simulink model "transfer_function_calculation"  (R2016a)
settings: Solver=VariableStepAuto  StartTime=0.0  StopTime=5  RelTol=1e-3
values from neighbouring files (symbols this model uses):
  a = .7    (= 0.7)    [PM_1_5MW_syn_27.m]
  Flux = 5.8264    [PM_1_5MW_syn_27.m]
  Id_set = 500    [PM_1_5MW_syn_27.m]
  Iq_set = -2200    [PM_1_5MW_syn_27.m]
  L = .0001    (= 0.0001)    [PM_1_5MW_syn_27.m]
  Ld = 0.001575    [PM_1_5MW_syn_27.m]
  Lq = 0.001575    [PM_1_5MW_syn_27.m]
  mn = 60000    [PM_1_5MW_syn_27.m]
  p = 26    [PM_1_5MW_syn_27.m]
  Rs = 0.000821    [PM_1_5MW_syn_27.m]
  Sollkurve_M_Optimum = [0 57121 101549 158670 228485 310994 406196 514092 634681 767965 810425 823386 ... (13 elements, 13x1)]    [Lookup_M_n.mat]
  Sollkurve_nGen_Optimum = [0 5 7 9 11 12 14 16 18 20 20.07 20.2 ... (13 elements, 13x1)]    [Lookup_M_n.mat]
  Speed_set = w_m    (= 2.10172548525)    [PM_1_5MW_syn_27.m]
  Ts_Power = 5.000000000000000e-06    (= 5e-06)    [PM_1_5MW_syn_27.m]
  Vdc = 1200    [PM_1_5MW_syn_27.m]
  Vh = Vm/6*0    (= 0)    [PM_1_5MW_syn_27.m]
undefined symbols (not defined in the file or in its folder): C2, Esw_Erec, Esw_Off, Esw_On, Page_Temp_C
undefined symbols (not defined in the file): Ts_Control, z
libraries: fl_lib x84, powerlib_meascontrol x58, simulink x56, nesl_utility x36, powerlib x33, simulink_extras x11
(part 2 of 6)

== system transfer_function_calculation/Generator/3 Level Converter2/Loss Calculation ==
  In1 : Inport
  In2 : Inport  Port=2
  In3 : Inport  Port=3
  In4 : Inport  Port=4
  In5 : Inport  Port=5
  In6 : Inport  Port=6
  In7 : Inport  Port=7
  In8 : Inport  Port=8
  In9 : Inport  Port=9
  In10 : Inport  Port=10
  In11 : Inport  Port=11
  In12 : Inport  Port=12
  "A;B;C phase losses " : Scope  NumInputPorts=4
  Leg A1 : Subsystem  mask(Half-Bridge IGBT with thermal model & losses calculation){Ron=1e-3, Rs=1e6, Cs=Inf, Tj_Init=123, PulseDuration=z, Ts=Ts_Power, Ts_Simscape=Ts_Control, IGBT_Rth_jc=0.051/10, IGBT_Cth_j=1.6804*2, IGBT_Vcc_Eon=1200, IGBT_Tj_Eon=[125 150], IGBT_Eon=[150 200 300 450 600 700 900 1000 1200 1400; 150 220 300 500 700 800 1000 1200 1400 1500], IGBT_Ic_Eon=[0 400 800 1600 2400 3200 4000 4800 5600 6400], IGBT_Vcc_Eoff=1200, IGBT_Tj_Eoff=[125 150], IGBT_Eoff=[150 200 400 610 950 1220 1600 2100 2600 3200; 200 350 570 900 1000 1300 1700 2100 2700 3400], IGBT_Ic_Eoff=[0 400 800 1600 2400 3200 4000 4800 5600 6400], IGBT_Tj_OnState=[125 150], IGBT_Vce_OnState=[.5 .81 .9 1 1.5 2 2.5 3 3.5; 0 0.5 .9 1 1.5 2.1 2.6 3.2 3.7], IGBT_Ic_OnState=[0 250 300 400 1300 2600 4200 5600 7200], DIODE_Rth_jc=0.102/10, DIODE_Cth_j=1.3235*2, DIODE_Vcc_Erec=1200, DIODE_Tj_Erec=[125 150], DIODE_Erec=[150 500 650 800 950 1050 1120 1190 1210;350 550 790 950 1100 1200 1270 1320 1350], DIODE_If_Erec=[0 900 1800 2700 3600 4500 5400 6300 7200], DIODE_Tj_OnState=[125 150], DIODE_Vf_OnState=[0 1.0 1.2 1.4 1.7 1.8 1.9 2.2 2.4 2.7;0 1 1.25 1.47 1.72 1.9 2 2.3 2.6 2.8], DIODE_If_OnState=[0 600 1200 1800 2400 3000 3600 4800 6000 7200]}
      mask prompts: Ron "Internal resistance Ron (Ohms):"; Rs "Snubber resistance (Ohms):"; Cs "Snubber capacitance (F):"; Tj_Init "Initial Junction Temperature (degrees Celsius):"; PulseDuration "Pulse Duration for Energy-to-Power conversion (s):"; Ts "Simscape Power Systems Sample Time (as specified in the Powergui) (s):"; Ts_Simscape "Simscape Solver Sample Time (s):"; IGBT_Rth_jc "Junction-to-Case thermal resistance (K/W):"; IGBT_Cth_j "Junction thermal capacitance (Joule/Kelvin):"; IGBT_Vcc_Eon "Vcc (V):"; IGBT_Tj_Eon "Tj  (Celsius):"; IGBT_Eon "Eon (V):"; IGBT_Ic_Eon "Ic (A):"; IGBT_Vcc_Eoff "Vcc (V):"; IGBT_Tj_Eoff "Tj (Celsius):"; IGBT_Eoff "Eoff (V):"; IGBT_Ic_Eoff "Ic (A):"; IGBT_Tj_OnState "Tj (Celsius):"; IGBT_Vce_OnState "Vce (V):"; IGBT_Ic_OnState "Ic (A):"; DIODE_Rth_jc "Junction-to-Case thermal resistance (K/W):"; DIODE_Cth_j "Junction thermal capacitance (Joule/Kelvin):"; DIODE_Vcc_Erec "Vcc (V):"; DIODE_Tj_Erec "Tj  (Celsius):"; DIODE_Erec "Erec (V):"; DIODE_If_Erec "If (A):"; DIODE_Tj_OnState "Tj (Celsius):"; DIODE_Vf_OnState "Vf (V):"; DIODE_If_OnState "If (A):"
      mask help: The half-bridge is modeled by two IGBT/Diode blocks. The upper and lower IGBT/Diode blocks are pulsed from an external pulse generator.
      mask init:
      | BlockName=gcb;
      | Tj0=Tj_Init;
      | 
      | % Add a row with 0 values for Eon and Eoff
      | E0_On=zeros(1,length(IGBT_Eon));
      | Esw_On(:,:,1)=[E0_On;IGBT_Eon(1,:)];
      | Esw_On(:,:,2)=[E0_On;IGBT_Eon(2,:)];
      | E0_Off=zeros(1,length(IGBT_Eoff));
      | Esw_Off(:,:,1)=[E0_Off;IGBT_Eoff(1,:)];
      | Esw_Off(:,:,2)=[E0_Off;IGBT_Eoff(2,:)];
      | 
      | % Create a two-element vector for Vcc (first value = 0)
      | Vcc_Esw_On=[0 IGBT_Vcc_Eon];
      | Vcc_Esw_Off=[0 IGBT_Vcc_Eoff];
      | 
      | % Add a row with 0 values for Erec
      | E0_Erec=zeros(1,length(DIODE_Erec));
      | Esw_Erec(:,:,1)=[E0_Erec;DIODE_Erec(1,:)];
      | Esw_Erec(:,:,2)=[E0_Erec;DIODE_Erec(2,:)];
      | 
      | % Create a two-element vector for Vcc (first value = 0)
      | Vcc_Esw_Erec=[0 DIODE_Vcc_Erec];
      mask DialogControl Container7 Prompt: Specifications
      mask DialogControl Container8 Prompt: Turn-on switching energies
      mask DialogControl Container9 Prompt: Turn-off switching energies
      mask DialogControl Container10 Prompt: On-state characteristics
      mask DialogControl Control4 Prompt: Plot characteristics
      mask DialogControl Control4 Callback:
      | %
      | IGBT_Vcc_Eon = getSPSmaskvalues(gcb,{'IGBT_Vcc_Eon'});
      | IGBT_Tj_Eon  = getSPSmaskvalues(gcb,{'IGBT_Tj_Eon'});
      | IGBT_Eon     = getSPSmaskvalues(gcb,{'IGBT_Eon'});
      | IGBT_Ic_Eon  = getSPSmaskvalues(gcb,{'IGBT_Ic_Eon'});
      | %
      | IGBT_Vcc_Eoff = getSPSmaskvalues(gcb,{'IGBT_Vcc_Eoff'});
      | IGBT_Tj_Eoff  = getSPSmaskvalues(gcb,{'IGBT_Tj_Eoff'});
      | IGBT_Eoff     = getSPSmaskvalues(gcb,{'IGBT_Eoff'});
      | IGBT_Ic_Eoff  = getSPSmaskvalues(gcb,{'IGBT_Ic_Eoff'});
      | %
      | IGBT_Tj_OnState  = getSPSmaskvalues(gcb,{'IGBT_Tj_OnState'});
      | IGBT_Vce_OnState = getSPSmaskvalues(gcb,{'IGBT_Vce_OnState'});
      | IGBT_Ic_OnState  = getSPSmaskvalues(gcb,{'IGBT_Ic_OnState'});
      | %
      | h1=figure;
      | ScreenS=get(0,'Screensize');
      | set(h1,'Position',[ScreenS(3)/60 ScreenS(4)/12 ScreenS(3)/2.4 ScreenS(4)/1.25])
      | subplot(3,1,1)
      | plot(IGBT_Ic_Eon,IGBT_Eon(1,:),'blue', ...
      |      IGBT_Ic_Eon,IGBT_Eon(2,:),'red')
      | legend([num2str(IGBT_Tj_Eon(1)),' deg. C'],[num2str(IGBT_Tj_Eon(2)),' deg. C'],'Location','NorthWest')
      | grid
      | Vcc_Value= num2str(IGBT_Vcc_Eon,'%5.0f');
      | title(['IGBT Turn-on Switching Energy (Vcc= ', Vcc_Value, ' V)' ])
      | ylabel('Eon (mJ)')
      | xlabel('Ic (A)')
      | hold on
      | %
      | subplot(3,1,2)
      | plot(IGBT_Ic_Eoff,IGBT_Eoff(1,:),'blue', ...
      |     IGBT_Ic_Eoff,IGBT_Eoff(2,:),'red')
      | legend([num2str(IGBT_Tj_Eoff(1)),' deg. C'],[num2str(IGBT_Tj_Eoff(2)),' deg. C'],'Location','NorthWest')
      | grid
      | Vcc_Value= num2str(IGBT_Vcc_Eoff,'%5.0f');
      | title(['IGBT Turn-off Switching Energy (Vcc= ', Vcc_Value, ' V)' ])
      | ylabel('Eoff (mJ)')
      | xlabel('Ic (A)')
      | %
      | subplot(3,1,3)
      | plot(IGBT_Vce_OnState(1,:),IGBT_Ic_OnState,'blue', ...
      |     IGBT_Vce_OnState(2,:),IGBT_Ic_OnState,'red')
      | legend([num2str(IGBT_Tj_OnState(1)),' deg. C'],[num2str(IGBT_Tj_OnState(2)),' deg. C'],'Location','NorthWest')
      | grid
      | title('IGBT On-state Characteristics')
      | ylabel('Ic (A)')
      | xlabel('Vce (V)')
      mask DialogControl Container7_copy Prompt: Specifications
      mask DialogControl Container12 Prompt: Reverse recovery energy
      mask DialogControl Container13 Prompt: On-state characteristics
      mask DialogControl Control4_copy Prompt: Plot characteristics
      mask DialogControl Control4_copy Callback:
      | DIODE_If_Erec    = getSPSmaskvalues(gcb,{'DIODE_If_Erec'});
      | DIODE_Erec       = getSPSmaskvalues(gcb,{'DIODE_Erec'});
      | DIODE_Vcc_Erec   = getSPSmaskvalues(gcb,{'DIODE_Vcc_Erec'});
      | DIODE_Vf_OnState = getSPSmaskvalues(gcb,{'DIODE_Vf_OnState'});
      | DIODE_If_OnState = getSPSmaskvalues(gcb,{'DIODE_If_OnState'});
      | 
      | h2=figure;
      | ScreenS=get(0,'Screensize');
      | set(h2,'Position',[ScreenS(3)/2.3 ScreenS(4)/12 ScreenS(3)/2.4 ScreenS(4)/1.25])
      | subplot(2,1,1)
      | plot(DIODE_If_Erec,DIODE_Erec(1,:),'blue', ...
      |     DIODE_If_Erec,DIODE_Erec(2,:),'red')
      | legend('25 deg. C','125 deg. C','Location','NorthWest')
      | grid
      | Vcc_Value= num2str(DIODE_Vcc_Erec,'%5.0f');
      | title(['Diode Reverse Recovery Energy (Vcc= ', Vcc_Value, ' V)' ])
      | ylabel('Erec (mJ)')
      | xlabel('If (A)')
      | %
      | subplot(2,1,2)
      | plot(DIODE_Vf_OnState(1,:),DIODE_If_OnState,'blue', ...
      |     DIODE_Vf_OnState(2,:),DIODE_If_OnState,'red')
      | legend('25 deg. C','125 deg. C','Location','NorthWest')
      | grid
      | title('Diode On-state Characteristics')
      | ylabel('If (A)')
      | xlabel('Vf (V)')
      mask Display: image('C:\Users\Test\Desktop\inverter losses\loss.jpg');
  Leg A2 : Subsystem  mask(Half-Bridge IGBT with thermal model & losses calculation){Ron=1e-3, Rs=1e6, Cs=Inf, Tj_Init=123, PulseDuration=z, Ts=Ts_Power, Ts_Simscape=Ts_Control, IGBT_Rth_jc=0.051, IGBT_Cth_j=2.6804, IGBT_Vcc_Eon=1800, IGBT_Tj_Eon=[125 150], IGBT_Eon=[150 200 300 450 600 700 900 1000 1200 1400; 150 220 300 500 700 800 1000 1200 1400 1500], IGBT_Ic_Eon=[0 400 800 1600 2400 3200 4000 4800 5600 6400], IGBT_Vcc_Eoff=1800, IGBT_Tj_Eoff=[125 150], IGBT_Eoff=[150 200 400 610 950 1220 1600 2100 2600 3200; 200 350 570 900 1000 1300 1700 2100 2700 3400], IGBT_Ic_Eoff=[0 400 800 1600 2400 3200 4000 4800 5600 6400], IGBT_Tj_OnState=[125 150], IGBT_Vce_OnState=[.5 .81 .9 1 1.5 2 2.5 3 3.5; 0 0.5 .9 1 1.5 2.1 2.6 3.2 3.7], IGBT_Ic_OnState=[0 250 300 400 1300 2600 4200 5600 7200], DIODE_Rth_jc=0.102, DIODE_Cth_j=1.3235, DIODE_Vcc_Erec=1200, DIODE_Tj_Erec=[125 150], DIODE_Erec=[150 500 650 800 950 1050 1120 1190 1210;350 550 790 950 1100 1200 1270 1320 1350], DIODE_If_Erec=[0 900 1800 2700 3600 4500 5400 6300 7200], DIODE_Tj_OnState=[125 150], DIODE_Vf_OnState=[0 1.0 1.2 1.4 1.7 1.8 1.9 2.2 2.4 2.7;0 1 1.25 1.47 1.72 1.9 2 2.3 2.6 2.8], DIODE_If_OnState=[0 600 1200 1800 2400 3000 3600 4800 6000 7200]}
      mask prompts: Ron "Internal resistance Ron (Ohms):"; Rs "Snubber resistance (Ohms):"; Cs "Snubber capacitance (F):"; Tj_Init "Initial Junction Temperature (degrees Celsius):"; PulseDuration "Pulse Duration for Energy-to-Power conversion (s):"; Ts "Simscape Power Systems Sample Time (as specified in the Powergui) (s):"; Ts_Simscape "Simscape Solver Sample Time (s):"; IGBT_Rth_jc "Junction-to-Case thermal resistance (K/W):"; IGBT_Cth_j "Junction thermal capacitance (Joule/Kelvin):"; IGBT_Vcc_Eon "Vcc (V):"; IGBT_Tj_Eon "Tj  (Celsius):"; IGBT_Eon "Eon (V):"; IGBT_Ic_Eon "Ic (A):"; IGBT_Vcc_Eoff "Vcc (V):"; IGBT_Tj_Eoff "Tj (Celsius):"; IGBT_Eoff "Eoff (V):"; IGBT_Ic_Eoff "Ic (A):"; IGBT_Tj_OnState "Tj (Celsius):"; IGBT_Vce_OnState "Vce (V):"; IGBT_Ic_OnState "Ic (A):"; DIODE_Rth_jc "Junction-to-Case thermal resistance (K/W):"; DIODE_Cth_j "Junction thermal capacitance (Joule/Kelvin):"; DIODE_Vcc_Erec "Vcc (V):"; DIODE_Tj_Erec "Tj  (Celsius):"; DIODE_Erec "Erec (V):"; DIODE_If_Erec "If (A):"; DIODE_Tj_OnState "Tj (Celsius):"; DIODE_Vf_OnState "Vf (V):"; DIODE_If_OnState "If (A):"
      mask help: The half-bridge is modeled by two IGBT/Diode blocks. The upper and lower IGBT/Diode blocks are pulsed from an external pulse generator.
      mask init: same as transfer_function_calculation/Generator/3 Level Converter2/Loss Calculation/Leg A1
      mask DialogControl Container7 Prompt: Specifications
      mask DialogControl Container8 Prompt: Turn-on switching energies
      mask DialogControl Container9 Prompt: Turn-off switching energies
      mask DialogControl Container10 Prompt: On-state characteristics
      mask DialogControl Control4 Prompt: Plot characteristics
      mask DialogControl Control4 Callback:
      | %
      | IGBT_Vcc_Eon = getSPSmaskvalues(gcb,{'IGBT_Vcc_Eon'});
      | IGBT_Tj_Eon  = getSPSmaskvalues(gcb,{'IGBT_Tj_Eon'});
      | IGBT_Eon     = getSPSmaskvalues(gcb,{'IGBT_Eon'});
      | IGBT_Ic_Eon  = getSPSmaskvalues(gcb,{'IGBT_Ic_Eon'});
      | %
      | IGBT_Vcc_Eoff = getSPSmaskvalues(gcb,{'IGBT_Vcc_Eoff'});
      | IGBT_Tj_Eoff  = getSPSmaskvalues(gcb,{'IGBT_Tj_Eoff'});
      | IGBT_Eoff     = getSPSmaskvalues(gcb,{'IGBT_Eoff'});
      | IGBT_Ic_Eoff  = getSPSmaskvalues(gcb,{'IGBT_Ic_Eoff'});
      | %
      | IGBT_Tj_OnState  = getSPSmaskvalues(gcb,{'IGBT_Tj_OnState'});
      | IGBT_Vce_OnState = getSPSmaskvalues(gcb,{'IGBT_Vce_OnState'});
      | IGBT_Ic_OnState  = getSPSmaskvalues(gcb,{'IGBT_Ic_OnState'});
      | %
      | h1=figure;
      | ScreenS=get(0,'Screensize');
      | set(h1,'Position',[ScreenS(3)/60 ScreenS(4)/12 ScreenS(3)/2.4 ScreenS(4)/1.25])
      | subplot(3,1,1)
      | plot(IGBT_Ic_Eon,IGBT_Eon(1,:),'blue', ...
      |      IGBT_Ic_Eon,IGBT_Eon(2,:),'red')
      | legend([num2str(IGBT_Tj_Eon(1)),' deg. C'],[num2str(IGBT_Tj_Eon(2)),' deg. C'],'Location','NorthWest')
      | grid
      | Vcc_Value= num2str(IGBT_Vcc_Eon,'%5.0f');
      | title(['IGBT Turn-on Switching Energy (Vcc= ', Vcc_Value, ' V)' ])
      | ylabel('Eon (mJ)')
      | xlabel('Ic (A)')
      | hold on
      | %
      | subplot(3,1,2)
      | plot(IGBT_Ic_Eoff,IGBT_Eoff(1,:),'blue', ...
      |     IGBT_Ic_Eoff,IGBT_Eoff(2,:),'red')
      | legend([num2str(IGBT_Tj_Eoff(1)),' deg. C'],[num2str(IGBT_Tj_Eoff(2)),' deg. C'],'Location','NorthWest')
      | grid
      | Vcc_Value= num2str(IGBT_Vcc_Eoff,'%5.0f');
      | title(['IGBT Turn-off Switching Energy (Vcc= ', Vcc_Value, ' V)' ])
      | ylabel('Eoff (mJ)')
      | xlabel('Ic (A)')
      | %
      | subplot(3,1,3)
      | plot(IGBT_Vce_OnState(1,:),IGBT_Ic_OnState,'blue', ...
      |     IGBT_Vce_OnState(2,:),IGBT_Ic_OnState,'red')
      | legend([num2str(IGBT_Tj_OnState(1)),' deg. C'],[num2str(IGBT_Tj_OnState(2)),' deg. C'],'Location','NorthWest')
      | grid
      | title('IGBT On-state Characteristics')
      | ylabel('Ic (A)')
      | xlabel('Vce (V)')
      mask DialogControl Container7_copy Prompt: Specifications
      mask DialogControl Container12 Prompt: Reverse recovery energy
      mask DialogControl Container13 Prompt: On-state characteristics
      mask DialogControl Control4_copy Prompt: Plot characteristics
      mask DialogControl Control4_copy Callback:
      | DIODE_If_Erec    = getSPSmaskvalues(gcb,{'DIODE_If_Erec'});
      | DIODE_Erec       = getSPSmaskvalues(gcb,{'DIODE_Erec'});
      | DIODE_Vcc_Erec   = getSPSmaskvalues(gcb,{'DIODE_Vcc_Erec'});
      | DIODE_Vf_OnState = getSPSmaskvalues(gcb,{'DIODE_Vf_OnState'});
      | DIODE_If_OnState = getSPSmaskvalues(gcb,{'DIODE_If_OnState'});
      | 
      | h2=figure;
      | ScreenS=get(0,'Screensize');
      | set(h2,'Position',[ScreenS(3)/2.3 ScreenS(4)/12 ScreenS(3)/2.4 ScreenS(4)/1.25])
      | subplot(2,1,1)
      | plot(DIODE_If_Erec,DIODE_Erec(1,:),'blue', ...
      |     DIODE_If_Erec,DIODE_Erec(2,:),'red')
      | legend('25 deg. C','125 deg. C','Location','NorthWest')
      | grid
      | Vcc_Value= num2str(DIODE_Vcc_Erec,'%5.0f');
      | title(['Diode Reverse Recovery Energy (Vcc= ', Vcc_Value, ' V)' ])
      | ylabel('Erec (mJ)')
      | xlabel('If (A)')
      | %
      | subplot(2,1,2)
      | plot(DIODE_Vf_OnState(1,:),DIODE_If_OnState,'blue', ...
      |     DIODE_Vf_OnState(2,:),DIODE_If_OnState,'red')
      | legend('25 deg. C','125 deg. C','Location','NorthWest')
      | grid
      | title('Diode On-state Characteristics')
      | ylabel('If (A)')
      | xlabel('Vf (V)')
      mask Display: image('C:\Users\Test\Desktop\inverter losses\loss.jpg');
  Leg B1 : Subsystem  mask(Half-Bridge IGBT with thermal model & losses calculation){Ron=1e-3, Rs=1e6, Cs=Inf, Tj_Init=123, PulseDuration=z, Ts=Ts_Power, Ts_Simscape=Ts_Control, IGBT_Rth_jc=0.051, IGBT_Cth_j=2.6804, IGBT_Vcc_Eon=1200, IGBT_Tj_Eon=[125 150], IGBT_Eon=[150 200 300 450 600 700 900 1000 1200 1400; 150 220 300 500 700 800 1000 1200 1400 1500], IGBT_Ic_Eon=[0 400 800 1600 2400 3200 4000 4800 5600 6400], IGBT_Vcc_Eoff=1200, IGBT_Tj_Eoff=[125 150], IGBT_Eoff=[150 200 400 610 950 1220 1600 2100 2600 3200; 200 350 570 900 1000 1300 1700 2100 2700 3400], IGBT_Ic_Eoff=[0 400 800 1600 2400 3200 4000 4800 5600 6400], IGBT_Tj_OnState=[125 150], IGBT_Vce_OnState=[.5 .81 .9 1 1.5 2 2.5 3 3.5; 0 0.5 .9 1 1.5 2.1 2.6 3.2 3.7], IGBT_Ic_OnState=[0 250 300 400 1300 2600 4200 5600 7200], DIODE_Rth_jc=0.102, DIODE_Cth_j=1.3235, DIODE_Vcc_Erec=1200, DIODE_Tj_Erec=[125 150], DIODE_Erec=[150 500 650 800 950 1050 1120 1190 1210;350 550 790 950 1100 1200 1270 1320 1350], DIODE_If_Erec=[0 900 1800 2700 3600 4500 5400 6300 7200], DIODE_Tj_OnState=[125 150], DIODE_Vf_OnState=[0 1.0 1.2 1.4 1.7 1.8 1.9 2.2 2.4 2.7;0 1 1.25 1.47 1.72 1.9 2 2.3 2.6 2.8], DIODE_If_OnState=[0 600 1200 1800 2400 3000 3600 4800 6000 7200]}
      mask prompts: Ron "Internal resistance Ron (Ohms):"; Rs "Snubber resistance (Ohms):"; Cs "Snubber capacitance (F):"; Tj_Init "Initial Junction Temperature (degrees Celsius):"; PulseDuration "Pulse Duration for Energy-to-Power conversion (s):"; Ts "Simscape Power Systems Sample Time (as specified in the Powergui) (s):"; Ts_Simscape "Simscape Solver Sample Time (s):"; IGBT_Rth_jc "Junction-to-Case thermal resistance (K/W):"; IGBT_Cth_j "Junction thermal capacitance (Joule/Kelvin):"; IGBT_Vcc_Eon "Vcc (V):"; IGBT_Tj_Eon "Tj  (Celsius):"; IGBT_Eon "Eon (V):"; IGBT_Ic_Eon "Ic (A):"; IGBT_Vcc_Eoff "Vcc (V):"; IGBT_Tj_Eoff "Tj (Celsius):"; IGBT_Eoff "Eoff (V):"; IGBT_Ic_Eoff "Ic (A):"; IGBT_Tj_OnState "Tj (Celsius):"; IGBT_Vce_OnState "Vce (V):"; IGBT_Ic_OnState "Ic (A):"; DIODE_Rth_jc "Junction-to-Case thermal resistance (K/W):"; DIODE_Cth_j "Junction thermal capacitance (Joule/Kelvin):"; DIODE_Vcc_Erec "Vcc (V):"; DIODE_Tj_Erec "Tj  (Celsius):"; DIODE_Erec "Erec (V):"; DIODE_If_Erec "If (A):"; DIODE_Tj_OnState "Tj (Celsius):"; DIODE_Vf_OnState "Vf (V):"; DIODE_If_OnState "If (A):"
      mask help: The half-bridge is modeled by two IGBT/Diode blocks. The upper and lower IGBT/Diode blocks are pulsed from an external pulse generator.
      mask init: same as transfer_function_calculation/Generator/3 Level Converter2/Loss Calculation/Leg A1
      mask DialogControl Container7 Prompt: Specifications
      mask DialogControl Container8 Prompt: Turn-on switching energies
      mask DialogControl Container9 Prompt: Turn-off switching energies
      mask DialogControl Container10 Prompt: On-state characteristics
      mask DialogControl Control4 Prompt: Plot characteristics
      mask DialogControl Control4 Callback:
      | %
      | IGBT_Vcc_Eon = getSPSmaskvalues(gcb,{'IGBT_Vcc_Eon'});
      | IGBT_Tj_Eon  = getSPSmaskvalues(gcb,{'IGBT_Tj_Eon'});
      | IGBT_Eon     = getSPSmaskvalues(gcb,{'IGBT_Eon'});
      | IGBT_Ic_Eon  = getSPSmaskvalues(gcb,{'IGBT_Ic_Eon'});
      | %
      | IGBT_Vcc_Eoff = getSPSmaskvalues(gcb,{'IGBT_Vcc_Eoff'});
      | IGBT_Tj_Eoff  = getSPSmaskvalues(gcb,{'IGBT_Tj_Eoff'});
      | IGBT_Eoff     = getSPSmaskvalues(gcb,{'IGBT_Eoff'});
      | IGBT_Ic_Eoff  = getSPSmaskvalues(gcb,{'IGBT_Ic_Eoff'});
      | %
      | IGBT_Tj_OnState  = getSPSmaskvalues(gcb,{'IGBT_Tj_OnState'});
      | IGBT_Vce_OnState = getSPSmaskvalues(gcb,{'IGBT_Vce_OnState'});
      | IGBT_Ic_OnState  = getSPSmaskvalues(gcb,{'IGBT_Ic_OnState'});
      | %
      | h1=figure;
      | ScreenS=get(0,'Screensize');
      | set(h1,'Position',[ScreenS(3)/60 ScreenS(4)/12 ScreenS(3)/2.4 ScreenS(4)/1.25])
      | subplot(3,1,1)
      | plot(IGBT_Ic_Eon,IGBT_Eon(1,:),'blue', ...
      |      IGBT_Ic_Eon,IGBT_Eon(2,:),'red')
      | legend([num2str(IGBT_Tj_Eon(1)),' deg. C'],[num2str(IGBT_Tj_Eon(2)),' deg. C'],'Location','NorthWest')
      | grid
      | Vcc_Value= num2str(IGBT_Vcc_Eon,'%5.0f');
      | title(['IGBT Turn-on Switching Energy (Vcc= ', Vcc_Value, ' V)' ])
      | ylabel('Eon (mJ)')
      | xlabel('Ic (A)')
      | hold on
      | %
      | subplot(3,1,2)
      | plot(IGBT_Ic_Eoff,IGBT_Eoff(1,:),'blue', ...
      |     IGBT_Ic_Eoff,IGBT_Eoff(2,:),'red')
      | legend([num2str(IGBT_Tj_Eoff(1)),' deg. C'],[num2str(IGBT_Tj_Eoff(2)),' deg. C'],'Location','NorthWest')
      | grid
      | Vcc_Value= num2str(IGBT_Vcc_Eoff,'%5.0f');
      | title(['IGBT Turn-off Switching Energy (Vcc= ', Vcc_Value, ' V)' ])
      | ylabel('Eoff (mJ)')
      | xlabel('Ic (A)')
      | %
      | subplot(3,1,3)
      | plot(IGBT_Vce_OnState(1,:),IGBT_Ic_OnState,'blue', ...
      |     IGBT_Vce_OnState(2,:),IGBT_Ic_OnState,'red')
      | legend([num2str(IGBT_Tj_OnState(1)),' deg. C'],[num2str(IGBT_Tj_OnState(2)),' deg. C'],'Location','NorthWest')
      | grid
      | title('IGBT On-state Characteristics')
      | ylabel('Ic (A)')
      | xlabel('Vce (V)')
      mask DialogControl Container7_copy Prompt: Specifications
      mask DialogControl Container12 Prompt: Reverse recovery energy
      mask DialogControl Container13 Prompt: On-state characteristics
      mask DialogControl Control4_copy Prompt: Plot characteristics
      mask DialogControl Control4_copy Callback:
      | DIODE_If_Erec    = getSPSmaskvalues(gcb,{'DIODE_If_Erec'});
      | DIODE_Erec       = getSPSmaskvalues(gcb,{'DIODE_Erec'});
      | DIODE_Vcc_Erec   = getSPSmaskvalues(gcb,{'DIODE_Vcc_Erec'});
      | DIODE_Vf_OnState = getSPSmaskvalues(gcb,{'DIODE_Vf_OnState'});
      | DIODE_If_OnState = getSPSmaskvalues(gcb,{'DIODE_If_OnState'});
      | 
      | h2=figure;
      | ScreenS=get(0,'Screensize');
      | set(h2,'Position',[ScreenS(3)/2.3 ScreenS(4)/12 ScreenS(3)/2.4 ScreenS(4)/1.25])
      | subplot(2,1,1)
      | plot(DIODE_If_Erec,DIODE_Erec(1,:),'blue', ...
      |     DIODE_If_Erec,DIODE_Erec(2,:),'red')
      | legend('25 deg. C','125 deg. C','Location','NorthWest')
      | grid
      | Vcc_Value= num2str(DIODE_Vcc_Erec,'%5.0f');
      | title(['Diode Reverse Recovery Energy (Vcc= ', Vcc_Value, ' V)' ])
      | ylabel('Erec (mJ)')
      | xlabel('If (A)')
      | %
      | subplot(2,1,2)
      | plot(DIODE_Vf_OnState(1,:),DIODE_If_OnState,'blue', ...
      |     DIODE_Vf_OnState(2,:),DIODE_If_OnState,'red')
      | legend('25 deg. C','125 deg. C','Location','NorthWest')
      | grid
      | title('Diode On-state Characteristics')
      | ylabel('If (A)')
      | xlabel('Vf (V)')
      mask Display: image('C:\Users\Test\Desktop\inverter losses\loss.jpg');
  Leg B2 : Subsystem  mask(Half-Bridge IGBT with thermal model & losses calculation){Ron=1e-3, Rs=1e6, Cs=Inf, Tj_Init=123, PulseDuration=z, Ts=Ts_Power, Ts_Simscape=Ts_Control, IGBT_Rth_jc=0.051, IGBT_Cth_j=2.6804, IGBT_Vcc_Eon=1200, IGBT_Tj_Eon=[125 150], IGBT_Eon=[150 200 300 450 600 700 900 1000 1200 1400; 150 220 300 500 700 800 1000 1200 1400 1500], IGBT_Ic_Eon=[0 400 800 1600 2400 3200 4000 4800 5600 6400], IGBT_Vcc_Eoff=1200, IGBT_Tj_Eoff=[125 150], IGBT_Eoff=[150 200 400 610 950 1220 1600 2100 2600 3200; 200 350 570 900 1000 1300 1700 2100 2700 3400], IGBT_Ic_Eoff=[0 400 800 1600 2400 3200 4000 4800 5600 6400], IGBT_Tj_OnState=[125 150], IGBT_Vce_OnState=[.5 .81 .9 1 1.5 2 2.5 3 3.5; 0 0.5 .9 1 1.5 2.1 2.6 3.2 3.7], IGBT_Ic_OnState=[0 250 300 400 1300 2600 4200 5600 7200], DIODE_Rth_jc=0.102, DIODE_Cth_j=1.3235, DIODE_Vcc_Erec=1200, DIODE_Tj_Erec=[125 150], DIODE_Erec=[150 500 650 800 950 1050 1120 1190 1210;350 550 790 950 1100 1200 1270 1320 1350], DIODE_If_Erec=[0 900 1800 2700 3600 4500 5400 6300 7200], DIODE_Tj_OnState=[125 150], DIODE_Vf_OnState=[0 1.0 1.2 1.4 1.7 1.8 1.9 2.2 2.4 2.7;0 1 1.25 1.47 1.72 1.9 2 2.3 2.6 2.8], DIODE_If_OnState=[0 600 1200 1800 2400 3000 3600 4800 6000 7200]}
      mask prompts: Ron "Internal resistance Ron (Ohms):"; Rs "Snubber resistance (Ohms):"; Cs "Snubber capacitance (F):"; Tj_Init "Initial Junction Temperature (degrees Celsius):"; PulseDuration "Pulse Duration for Energy-to-Power conversion (s):"; Ts "Simscape Power Systems Sample Time (as specified in the Powergui) (s):"; Ts_Simscape "Simscape Solver Sample Time (s):"; IGBT_Rth_jc "Junction-to-Case thermal resistance (K/W):"; IGBT_Cth_j "Junction thermal capacitance (Joule/Kelvin):"; IGBT_Vcc_Eon "Vcc (V):"; IGBT_Tj_Eon "Tj  (Celsius):"; IGBT_Eon "Eon (V):"; IGBT_Ic_Eon "Ic (A):"; IGBT_Vcc_Eoff "Vcc (V):"; IGBT_Tj_Eoff "Tj (Celsius):"; IGBT_Eoff "Eoff (V):"; IGBT_Ic_Eoff "Ic (A):"; IGBT_Tj_OnState "Tj (Celsius):"; IGBT_Vce_OnState "Vce (V):"; IGBT_Ic_OnState "Ic (A):"; DIODE_Rth_jc "Junction-to-Case thermal resistance (K/W):"; DIODE_Cth_j "Junction thermal capacitance (Joule/Kelvin):"; DIODE_Vcc_Erec "Vcc (V):"; DIODE_Tj_Erec "Tj  (Celsius):"; DIODE_Erec "Erec (V):"; DIODE_If_Erec "If (A):"; DIODE_Tj_OnState "Tj (Celsius):"; DIODE_Vf_OnState "Vf (V):"; DIODE_If_OnState "If (A):"
      mask help: The half-bridge is modeled by two IGBT/Diode blocks. The upper and lower IGBT/Diode blocks are pulsed from an external pulse generator.
      mask init: same as transfer_function_calculation/Generator/3 Level Converter2/Loss Calculation/Leg A1
      mask DialogControl Container7 Prompt: Specifications
      mask DialogControl Container8 Prompt: Turn-on switching energies
      mask DialogControl Container9 Prompt: Turn-off switching energies
      mask DialogControl Container10 Prompt: On-state characteristics
      mask DialogControl Control4 Prompt: Plot characteristics
      mask DialogControl Control4 Callback:
      | %
      | IGBT_Vcc_Eon = getSPSmaskvalues(gcb,{'IGBT_Vcc_Eon'});
      | IGBT_Tj_Eon  = getSPSmaskvalues(gcb,{'IGBT_Tj_Eon'});
      | IGBT_Eon     = getSPSmaskvalues(gcb,{'IGBT_Eon'});
      | IGBT_Ic_Eon  = getSPSmaskvalues(gcb,{'IGBT_Ic_Eon'});
      | %
      | IGBT_Vcc_Eoff = getSPSmaskvalues(gcb,{'IGBT_Vcc_Eoff'});
      | IGBT_Tj_Eoff  = getSPSmaskvalues(gcb,{'IGBT_Tj_Eoff'});
      | IGBT_Eoff     = getSPSmaskvalues(gcb,{'IGBT_Eoff'});
      | IGBT_Ic_Eoff  = getSPSmaskvalues(gcb,{'IGBT_Ic_Eoff'});
      | %
      | IGBT_Tj_OnState  = getSPSmaskvalues(gcb,{'IGBT_Tj_OnState'});
      | IGBT_Vce_OnState = getSPSmaskvalues(gcb,{'IGBT_Vce_OnState'});
      | IGBT_Ic_OnState  = getSPSmaskvalues(gcb,{'IGBT_Ic_OnState'});
      | %
      | h1=figure;
      | ScreenS=get(0,'Screensize');
      | set(h1,'Position',[ScreenS(3)/60 ScreenS(4)/12 ScreenS(3)/2.4 ScreenS(4)/1.25])
      | subplot(3,1,1)
      | plot(IGBT_Ic_Eon,IGBT_Eon(1,:),'blue', ...
      |      IGBT_Ic_Eon,IGBT_Eon(2,:),'red')
      | legend([num2str(IGBT_Tj_Eon(1)),' deg. C'],[num2str(IGBT_Tj_Eon(2)),' deg. C'],'Location','NorthWest')
      | grid
      | Vcc_Value= num2str(IGBT_Vcc_Eon,'%5.0f');
      | title(['IGBT Turn-on Switching Energy (Vcc= ', Vcc_Value, ' V)' ])
      | ylabel('Eon (mJ)')
      | xlabel('Ic (A)')
      | hold on
      | %
      | subplot(3,1,2)
      | plot(IGBT_Ic_Eoff,IGBT_Eoff(1,:),'blue', ...
      |     IGBT_Ic_Eoff,IGBT_Eoff(2,:),'red')
      | legend([num2str(IGBT_Tj_Eoff(1)),' deg. C'],[num2str(IGBT_Tj_Eoff(2)),' deg. C'],'Location','NorthWest')
      | grid
      | Vcc_Value= num2str(IGBT_Vcc_Eoff,'%5.0f');
      | title(['IGBT Turn-off Switching Energy (Vcc= ', Vcc_Value, ' V)' ])
      | ylabel('Eoff (mJ)')
      | xlabel('Ic (A)')
      | %
      | subplot(3,1,3)
      | plot(IGBT_Vce_OnState(1,:),IGBT_Ic_OnState,'blue', ...
      |     IGBT_Vce_OnState(2,:),IGBT_Ic_OnState,'red')
      | legend([num2str(IGBT_Tj_OnState(1)),' deg. C'],[num2str(IGBT_Tj_OnState(2)),' deg. C'],'Location','NorthWest')
      | grid
      | title('IGBT On-state Characteristics')
      | ylabel('Ic (A)')
      | xlabel('Vce (V)')
      mask DialogControl Container7_copy Prompt: Specifications
      mask DialogControl Container12 Prompt: Reverse recovery energy
      mask DialogControl Container13 Prompt: On-state characteristics
      mask DialogControl Control4_copy Prompt: Plot characteristics
      mask DialogControl Control4_copy Callback:
      | DIODE_If_Erec    = getSPSmaskvalues(gcb,{'DIODE_If_Erec'});
      | DIODE_Erec       = getSPSmaskvalues(gcb,{'DIODE_Erec'});
      | DIODE_Vcc_Erec   = getSPSmaskvalues(gcb,{'DIODE_Vcc_Erec'});
      | DIODE_Vf_OnState = getSPSmaskvalues(gcb,{'DIODE_Vf_OnState'});
      | DIODE_If_OnState = getSPSmaskvalues(gcb,{'DIODE_If_OnState'});
      | 
      | h2=figure;
      | ScreenS=get(0,'Screensize');
      | set(h2,'Position',[ScreenS(3)/2.3 ScreenS(4)/12 ScreenS(3)/2.4 ScreenS(4)/1.25])
      | subplot(2,1,1)
      | plot(DIODE_If_Erec,DIODE_Erec(1,:),'blue', ...
      |     DIODE_If_Erec,DIODE_Erec(2,:),'red')
      | legend('25 deg. C','125 deg. C','Location','NorthWest')
      | grid
      | Vcc_Value= num2str(DIODE_Vcc_Erec,'%5.0f');
      | title(['Diode Reverse Recovery Energy (Vcc= ', Vcc_Value, ' V)' ])
      | ylabel('Erec (mJ)')
      | xlabel('If (A)')
      | %
      | subplot(2,1,2)
      | plot(DIODE_Vf_OnState(1,:),DIODE_If_OnState,'blue', ...
      |     DIODE_Vf_OnState(2,:),DIODE_If_OnState,'red')
      | legend('25 deg. C','125 deg. C','Location','NorthWest')
      | grid
      | title('Diode On-state Characteristics')
      | ylabel('If (A)')
      | xlabel('Vf (V)')
      mask Display: image('C:\Users\Test\Desktop\inverter losses\loss.jpg');
  Leg C1 : Subsystem  mask(Half-Bridge IGBT with thermal model & losses calculation){Ron=1e-3, Rs=1e6, Cs=Inf, Tj_Init=123, PulseDuration=z, Ts=Ts_Power, Ts_Simscape=Ts_Control, IGBT_Rth_jc=0.051, IGBT_Cth_j=2.6804, IGBT_Vcc_Eon=1200, IGBT_Tj_Eon=[125 150], IGBT_Eon=[150 200 300 450 600 700 900 1000 1200 1400; 150 220 300 500 700 800 1000 1200 1400 1500], IGBT_Ic_Eon=[0 400 800 1600 2400 3200 4000 4800 5600 6400], IGBT_Vcc_Eoff=1200, IGBT_Tj_Eoff=[125 150], IGBT_Eoff=[150 200 400 610 950 1220 1600 2100 2600 3200; 200 350 570 900 1000 1300 1700 2100 2700 3400], IGBT_Ic_Eoff=[0 400 800 1600 2400 3200 4000 4800 5600 6400], IGBT_Tj_OnState=[125 150], IGBT_Vce_OnState=[.5 .81 .9 1 1.5 2 2.5 3 3.5; 0 0.5 .9 1 1.5 2.1 2.6 3.2 3.7], IGBT_Ic_OnState=[0 250 300 400 1300 2600 4200 5600 7200], DIODE_Rth_jc=0.102, DIODE_Cth_j=1.3235, DIODE_Vcc_Erec=1200, DIODE_Tj_Erec=[125 150], DIODE_Erec=[150 500 650 800 950 1050 1120 1190 1210;350 550 790 950 1100 1200 1270 1320 1350], DIODE_If_Erec=[0 900 1800 2700 3600 4500 5400 6300 7200], DIODE_Tj_OnState=[125 150], DIODE_Vf_OnState=[0 1.0 1.2 1.4 1.7 1.8 1.9 2.2 2.4 2.7;0 1 1.25 1.47 1.72 1.9 2 2.3 2.6 2.8], DIODE_If_OnState=[0 600 1200 1800 2400 3000 3600 4800 6000 7200]}
      mask prompts: Ron "Internal resistance Ron (Ohms):"; Rs "Snubber resistance (Ohms):"; Cs "Snubber capacitance (F):"; Tj_Init "Initial Junction Temperature (degrees Celsius):"; PulseDuration "Pulse Duration for Energy-to-Power conversion (s):"; Ts "Simscape Power Systems Sample Time (as specified in the Powergui) (s):"; Ts_Simscape "Simscape Solver Sample Time (s):"; IGBT_Rth_jc "Junction-to-Case thermal resistance (K/W):"; IGBT_Cth_j "Junction thermal capacitance (Joule/Kelvin):"; IGBT_Vcc_Eon "Vcc (V):"; IGBT_Tj_Eon "Tj  (Celsius):"; IGBT_Eon "Eon (V):"; IGBT_Ic_Eon "Ic (A):"; IGBT_Vcc_Eoff "Vcc (V):"; IGBT_Tj_Eoff "Tj (Celsius):"; IGBT_Eoff "Eoff (V):"; IGBT_Ic_Eoff "Ic (A):"; IGBT_Tj_OnState "Tj (Celsius):"; IGBT_Vce_OnState "Vce (V):"; IGBT_Ic_OnState "Ic (A):"; DIODE_Rth_jc "Junction-to-Case thermal resistance (K/W):"; DIODE_Cth_j "Junction thermal capacitance (Joule/Kelvin):"; DIODE_Vcc_Erec "Vcc (V):"; DIODE_Tj_Erec "Tj  (Celsius):"; DIODE_Erec "Erec (V):"; DIODE_If_Erec "If (A):"; DIODE_Tj_OnState "Tj (Celsius):"; DIODE_Vf_OnState "Vf (V):"; DIODE_If_OnState "If (A):"
      mask help: The half-bridge is modeled by two IGBT/Diode blocks. The upper and lower IGBT/Diode blocks are pulsed from an external pulse generator.
      mask init: same as transfer_function_calculation/Generator/3 Level Converter2/Loss Calculation/Leg A1
      mask DialogControl Container7 Prompt: Specifications
      mask DialogControl Container8 Prompt: Turn-on switching energies
      mask DialogControl Container9 Prompt: Turn-off switching energies
      mask DialogControl Container10 Prompt: On-state characteristics
      mask DialogControl Control4 Prompt: Plot characteristics
      mask DialogControl Control4 Callback:
      | %
      | IGBT_Vcc_Eon = getSPSmaskvalues(gcb,{'IGBT_Vcc_Eon'});
      | IGBT_Tj_Eon  = getSPSmaskvalues(gcb,{'IGBT_Tj_Eon'});
      | IGBT_Eon     = getSPSmaskvalues(gcb,{'IGBT_Eon'});
      | IGBT_Ic_Eon  = getSPSmaskvalues(gcb,{'IGBT_Ic_Eon'});
      | %
      | IGBT_Vcc_Eoff = getSPSmaskvalues(gcb,{'IGBT_Vcc_Eoff'});
      | IGBT_Tj_Eoff  = getSPSmaskvalues(gcb,{'IGBT_Tj_Eoff'});
      | IGBT_Eoff     = getSPSmaskvalues(gcb,{'IGBT_Eoff'});
      | IGBT_Ic_Eoff  = getSPSmaskvalues(gcb,{'IGBT_Ic_Eoff'});
      | %
      | IGBT_Tj_OnState  = getSPSmaskvalues(gcb,{'IGBT_Tj_OnState'});
      | IGBT_Vce_OnState = getSPSmaskvalues(gcb,{'IGBT_Vce_OnState'});
      | IGBT_Ic_OnState  = getSPSmaskvalues(gcb,{'IGBT_Ic_OnState'});
      | %
      | h1=figure;
      | ScreenS=get(0,'Screensize');
      | set(h1,'Position',[ScreenS(3)/60 ScreenS(4)/12 ScreenS(3)/2.4 ScreenS(4)/1.25])
      | subplot(3,1,1)
      | plot(IGBT_Ic_Eon,IGBT_Eon(1,:),'blue', ...
      |      IGBT_Ic_Eon,IGBT_Eon(2,:),'red')
      | legend([num2str(IGBT_Tj_Eon(1)),' deg. C'],[num2str(IGBT_Tj_Eon(2)),' deg. C'],'Location','NorthWest')
      | grid
      | Vcc_Value= num2str(IGBT_Vcc_Eon,'%5.0f');
      | title(['IGBT Turn-on Switching Energy (Vcc= ', Vcc_Value, ' V)' ])
      | ylabel('Eon (mJ)')
      | xlabel('Ic (A)')
      | hold on
      | %
      | subplot(3,1,2)
      | plot(IGBT_Ic_Eoff,IGBT_Eoff(1,:),'blue', ...
      |     IGBT_Ic_Eoff,IGBT_Eoff(2,:),'red')
      | legend([num2str(IGBT_Tj_Eoff(1)),' deg. C'],[num2str(IGBT_Tj_Eoff(2)),' deg. C'],'Location','NorthWest')
      | grid
      | Vcc_Value= num2str(IGBT_Vcc_Eoff,'%5.0f');
      | title(['IGBT Turn-off Switching Energy (Vcc= ', Vcc_Value, ' V)' ])
      | ylabel('Eoff (mJ)')
      | xlabel('Ic (A)')
      | %
      | subplot(3,1,3)
      | plot(IGBT_Vce_OnState(1,:),IGBT_Ic_OnState,'blue', ...
      |     IGBT_Vce_OnState(2,:),IGBT_Ic_OnState,'red')
      | legend([num2str(IGBT_Tj_OnState(1)),' deg. C'],[num2str(IGBT_Tj_OnState(2)),' deg. C'],'Location','NorthWest')
      | grid
      | title('IGBT On-state Characteristics')
      | ylabel('Ic (A)')
      | xlabel('Vce (V)')
      mask DialogControl Container7_copy Prompt: Specifications
      mask DialogControl Container12 Prompt: Reverse recovery energy
      mask DialogControl Container13 Prompt: On-state characteristics
      mask DialogControl Control4_copy Prompt: Plot characteristics
      mask DialogControl Control4_copy Callback:
      | DIODE_If_Erec    = getSPSmaskvalues(gcb,{'DIODE_If_Erec'});
      | DIODE_Erec       = getSPSmaskvalues(gcb,{'DIODE_Erec'});
      | DIODE_Vcc_Erec   = getSPSmaskvalues(gcb,{'DIODE_Vcc_Erec'});
      | DIODE_Vf_OnState = getSPSmaskvalues(gcb,{'DIODE_Vf_OnState'});
      | DIODE_If_OnState = getSPSmaskvalues(gcb,{'DIODE_If_OnState'});
      | 
      | h2=figure;
      | ScreenS=get(0,'Screensize');
      | set(h2,'Position',[ScreenS(3)/2.3 ScreenS(4)/12 ScreenS(3)/2.4 ScreenS(4)/1.25])
      | subplot(2,1,1)
      | plot(DIODE_If_Erec,DIODE_Erec(1,:),'blue', ...
      |     DIODE_If_Erec,DIODE_Erec(2,:),'red')
      | legend('25 deg. C','125 deg. C','Location','NorthWest')
      | grid
      | Vcc_Value= num2str(DIODE_Vcc_Erec,'%5.0f');
      | title(['Diode Reverse Recovery Energy (Vcc= ', Vcc_Value, ' V)' ])
      | ylabel('Erec (mJ)')
      | xlabel('If (A)')
      | %
      | subplot(2,1,2)
      | plot(DIODE_Vf_OnState(1,:),DIODE_If_OnState,'blue', ...
      |     DIODE_Vf_OnState(2,:),DIODE_If_OnState,'red')
      | legend('25 deg. C','125 deg. C','Location','NorthWest')
      | grid
      | title('Diode On-state Characteristics')
      | ylabel('If (A)')
      | xlabel('Vf (V)')
      mask Display: image('C:\Users\Test\Desktop\inverter losses\loss.jpg');
  Leg C2 : Subsystem  mask(Half-Bridge IGBT with thermal model & losses calculation){Ron=1e-3, Rs=1e6, Cs=Inf, Tj_Init=123, PulseDuration=z, Ts=Ts_Power, Ts_Simscape=Ts_Control, IGBT_Rth_jc=0.051, IGBT_Cth_j=2.6804, IGBT_Vcc_Eon=1200, IGBT_Tj_Eon=[125 150], IGBT_Eon=[150 200 300 450 600 700 900 1000 1200 1400; 150 220 300 500 700 800 1000 1200 1400 1500], IGBT_Ic_Eon=[0 400 800 1600 2400 3200 4000 4800 5600 6400], IGBT_Vcc_Eoff=1200, IGBT_Tj_Eoff=[125 150], IGBT_Eoff=[150 200 400 610 950 1220 1600 2100 2600 3200; 200 350 570 900 1000 1300 1700 2100 2700 3400], IGBT_Ic_Eoff=[0 400 800 1600 2400 3200 4000 4800 5600 6400], IGBT_Tj_OnState=[125 150], IGBT_Vce_OnState=[.5 .81 .9 1 1.5 2 2.5 3 3.5; 0 0.5 .9 1 1.5 2.1 2.6 3.2 3.7], IGBT_Ic_OnState=[0 250 300 400 1300 2600 4200 5600 7200], DIODE_Rth_jc=0.102, DIODE_Cth_j=1.3235, DIODE_Vcc_Erec=1200, DIODE_Tj_Erec=[125 150], DIODE_Erec=[150 500 650 800 950 1050 1120 1190 1210;350 550 790 950 1100 1200 1270 1320 1350], DIODE_If_Erec=[0 900 1800 2700 3600 4500 5400 6300 7200], DIODE_Tj_OnState=[125 150], DIODE_Vf_OnState=[0 1.0 1.2 1.4 1.7 1.8 1.9 2.2 2.4 2.7;0 1 1.25 1.47 1.72 1.9 2 2.3 2.6 2.8], DIODE_If_OnState=[0 600 1200 1800 2400 3000 3600 4800 6000 7200]}
      mask prompts: Ron "Internal resistance Ron (Ohms):"; Rs "Snubber resistance (Ohms):"; Cs "Snubber capacitance (F):"; Tj_Init "Initial Junction Temperature (degrees Celsius):"; PulseDuration "Pulse Duration for Energy-to-Power conversion (s):"; Ts "Simscape Power Systems Sample Time (as specified in the Powergui) (s):"; Ts_Simscape "Simscape Solver Sample Time (s):"; IGBT_Rth_jc "Junction-to-Case thermal resistance (K/W):"; IGBT_Cth_j "Junction thermal capacitance (Joule/Kelvin):"; IGBT_Vcc_Eon "Vcc (V):"; IGBT_Tj_Eon "Tj  (Celsius):"; IGBT_Eon "Eon (V):"; IGBT_Ic_Eon "Ic (A):"; IGBT_Vcc_Eoff "Vcc (V):"; IGBT_Tj_Eoff "Tj (Celsius):"; IGBT_Eoff "Eoff (V):"; IGBT_Ic_Eoff "Ic (A):"; IGBT_Tj_OnState "Tj (Celsius):"; IGBT_Vce_OnState "Vce (V):"; IGBT_Ic_OnState "Ic (A):"; DIODE_Rth_jc "Junction-to-Case thermal resistance (K/W):"; DIODE_Cth_j "Junction thermal capacitance (Joule/Kelvin):"; DIODE_Vcc_Erec "Vcc (V):"; DIODE_Tj_Erec "Tj  (Celsius):"; DIODE_Erec "Erec (V):"; DIODE_If_Erec "If (A):"; DIODE_Tj_OnState "Tj (Celsius):"; DIODE_Vf_OnState "Vf (V):"; DIODE_If_OnState "If (A):"
      mask help: The half-bridge is modeled by two IGBT/Diode blocks. The upper and lower IGBT/Diode blocks are pulsed from an external pulse generator.
      mask init: same as transfer_function_calculation/Generator/3 Level Converter2/Loss Calculation/Leg A1
      mask DialogControl Container7 Prompt: Specifications
      mask DialogControl Container8 Prompt: Turn-on switching energies
      mask DialogControl Container9 Prompt: Turn-off switching energies
      mask DialogControl Container10 Prompt: On-state characteristics
      mask DialogControl Control4 Prompt: Plot characteristics
      mask DialogControl Control4 Callback:
      | %
      | IGBT_Vcc_Eon = getSPSmaskvalues(gcb,{'IGBT_Vcc_Eon'});
      | IGBT_Tj_Eon  = getSPSmaskvalues(gcb,{'IGBT_Tj_Eon'});
      | IGBT_Eon     = getSPSmaskvalues(gcb,{'IGBT_Eon'});
      | IGBT_Ic_Eon  = getSPSmaskvalues(gcb,{'IGBT_Ic_Eon'});
      | %
      | IGBT_Vcc_Eoff = getSPSmaskvalues(gcb,{'IGBT_Vcc_Eoff'});
      | IGBT_Tj_Eoff  = getSPSmaskvalues(gcb,{'IGBT_Tj_Eoff'});
      | IGBT_Eoff     = getSPSmaskvalues(gcb,{'IGBT_Eoff'});
      | IGBT_Ic_Eoff  = getSPSmaskvalues(gcb,{'IGBT_Ic_Eoff'});
      | %
      | IGBT_Tj_OnState  = getSPSmaskvalues(gcb,{'IGBT_Tj_OnState'});
      | IGBT_Vce_OnState = getSPSmaskvalues(gcb,{'IGBT_Vce_OnState'});
      | IGBT_Ic_OnState  = getSPSmaskvalues(gcb,{'IGBT_Ic_OnState'});
      | %
      | h1=figure;
      | ScreenS=get(0,'Screensize');
      | set(h1,'Position',[ScreenS(3)/60 ScreenS(4)/12 ScreenS(3)/2.4 ScreenS(4)/1.25])
      | subplot(3,1,1)
      | plot(IGBT_Ic_Eon,IGBT_Eon(1,:),'blue', ...
      |      IGBT_Ic_Eon,IGBT_Eon(2,:),'red')
      | legend([num2str(IGBT_Tj_Eon(1)),' deg. C'],[num2str(IGBT_Tj_Eon(2)),' deg. C'],'Location','NorthWest')
      | grid
      | Vcc_Value= num2str(IGBT_Vcc_Eon,'%5.0f');
      | title(['IGBT Turn-on Switching Energy (Vcc= ', Vcc_Value, ' V)' ])
      | ylabel('Eon (mJ)')
      | xlabel('Ic (A)')
      | hold on
      | %
      | subplot(3,1,2)
      | plot(IGBT_Ic_Eoff,IGBT_Eoff(1,:),'blue', ...
      |     IGBT_Ic_Eoff,IGBT_Eoff(2,:),'red')
      | legend([num2str(IGBT_Tj_Eoff(1)),' deg. C'],[num2str(IGBT_Tj_Eoff(2)),' deg. C'],'Location','NorthWest')
      | grid
      | Vcc_Value= num2str(IGBT_Vcc_Eoff,'%5.0f');
      | title(['IGBT Turn-off Switching Energy (Vcc= ', Vcc_Value, ' V)' ])
      | ylabel('Eoff (mJ)')
      | xlabel('Ic (A)')
      | %
      | subplot(3,1,3)
      | plot(IGBT_Vce_OnState(1,:),IGBT_Ic_OnState,'blue', ...
      |     IGBT_Vce_OnState(2,:),IGBT_Ic_OnState,'red')
      | legend([num2str(IGBT_Tj_OnState(1)),' deg. C'],[num2str(IGBT_Tj_OnState(2)),' deg. C'],'Location','NorthWest')
      | grid
      | title('IGBT On-state Characteristics')
      | ylabel('Ic (A)')
      | xlabel('Vce (V)')
      mask DialogControl Container7_copy Prompt: Specifications
      mask DialogControl Container12 Prompt: Reverse recovery energy
      mask DialogControl Container13 Prompt: On-state characteristics
      mask DialogControl Control4_copy Prompt: Plot characteristics
      mask DialogControl Control4_copy Callback:
      | DIODE_If_Erec    = getSPSmaskvalues(gcb,{'DIODE_If_Erec'});
      | DIODE_Erec       = getSPSmaskvalues(gcb,{'DIODE_Erec'});
      | DIODE_Vcc_Erec   = getSPSmaskvalues(gcb,{'DIODE_Vcc_Erec'});
      | DIODE_Vf_OnState = getSPSmaskvalues(gcb,{'DIODE_Vf_OnState'});
      | DIODE_If_OnState = getSPSmaskvalues(gcb,{'DIODE_If_OnState'});
      | 
      | h2=figure;
      | ScreenS=get(0,'Screensize');
      | set(h2,'Position',[ScreenS(3)/2.3 ScreenS(4)/12 ScreenS(3)/2.4 ScreenS(4)/1.25])
      | subplot(2,1,1)
      | plot(DIODE_If_Erec,DIODE_Erec(1,:),'blue', ...
      |     DIODE_If_Erec,DIODE_Erec(2,:),'red')
      | legend('25 deg. C','125 deg. C','Location','NorthWest')
      | grid
      | Vcc_Value= num2str(DIODE_Vcc_Erec,'%5.0f');
      | title(['Diode Reverse Recovery Energy (Vcc= ', Vcc_Value, ' V)' ])
      | ylabel('Erec (mJ)')
      | xlabel('If (A)')
      | %
      | subplot(2,1,2)
      | plot(DIODE_Vf_OnState(1,:),DIODE_If_OnState,'blue', ...
      |     DIODE_Vf_OnState(2,:),DIODE_If_OnState,'red')
      | legend('25 deg. C','125 deg. C','Location','NorthWest')
      | grid
      | title('Diode On-state Characteristics')
      | ylabel('If (A)')
      | xlabel('Vf (V)')
      mask Display: image('C:\Users\Test\Desktop\inverter losses\loss.jpg');
  Phase A : Subsystem
  Phase B : Subsystem
  Phase C : Subsystem
  Scope : Scope  NumInputPorts=4
  Scope1 : Scope  NumInputPorts=4
  Scope2 : Scope  NumInputPorts=4
  Sum : Sum  Inputs=|+++
  Losses LegA : Outport
  Losses LegB : Outport  Port=2
  Losses LegC : Outport  Port=3
  Losses LegC1 : Outport  Port=4
  wires:
  In5/1 -> Leg B1/1(G)
  In4/1 -> Leg A2/2(G1)
  In9/1 -> Leg C1/1(G)
  In8/1 -> Leg B2/2(G1)
  In2/1 -> Leg A1/2(G1)
  In7/1 -> Leg B2/1(G)
  In1/1 -> Leg A1/1(G)
  In10/1 -> Leg C1/2(G1)
  In3/1 -> Leg A2/1(G)
  In12/1 -> Leg C2/2(G1)
  In11/1 -> Leg C2/1(G)
  In6/1 -> Leg B1/2(G1)
  Leg C1/1(m) -> Phase C/1(Leg C1)
  Leg B1/1(m) -> Phase B/1(Leg B1)
  Leg B2/1(m) -> Phase B/2(Leg B2)
  Leg C2/1(m) -> Phase C/2(Leg C2)
  Leg A1/1(m) -> Phase A/1(Leg A1)
  Leg A2/1(m) -> Phase A/2(Leg A2)
  Phase A/1(Losses LegA) -> Scope/1, Losses LegA/1
  Phase A/2(Tj  IGBTA1) -> Scope/2
  Phase A/3(Tj  IGBTA2) -> Scope/3
  Phase A/4(Tj  Case) -> Scope/4
  Phase B/1(Losses LegB) -> Scope1/1, Losses LegB/1
  Phase B/2(Tj  IGBTB1) -> Scope1/2
  Phase B/3(Tj  IGBTB2) -> Scope1/3
  Phase B/4(Tj  Case) -> Scope1/4
  Phase C/1(Losses LegC) -> Scope2/1, Losses LegC/1
  Phase C/2(Tj  IGBTC1) -> Scope2/2
  Phase C/3(Tj  IGBTC2) -> Scope2/3
  Phase C/4(Tj  Case) -> Scope2/4
  Phase A/5(Leg B) -> Sum/1, "A;B;C phase losses "/1
  Phase B/5(Leg A) -> Sum/2, "A;B;C phase losses "/2
  Phase C/5(Leg C) -> Sum/3, "A;B;C phase losses "/3
  Sum/1 -> "A;B;C phase losses "/4, Losses LegC1/1

== system transfer_function_calculation/Generator/3 Level Converter2/SPWM Generator ==
  A : Inport
  B : Inport  Port=2
  C : Inport  Port=3
  " Comparator Phase B" : Subsystem
  Comparator Phase A : Subsystem
  Comparator Phase C : Subsystem
  SPWM A : Subsystem
  SPWM B : Subsystem
  SPWM C : Subsystem
  Scope1 : Scope
  Scope2 : Scope
  Scope3 : Scope
  Scope4 : Scope  NumInputPorts=4
  Out1 : Outport
  Out2 : Outport  Port=2
  Out3 : Outport  Port=3
  Out4 : Outport  Port=4
  Out5 : Outport  Port=5
  Out6 : Outport  Port=6
  Out7 : Outport  Port=7
  Out8 : Outport  Port=8
  Out9 : Outport  Port=9
  Out10 : Outport  Port=10
  Out11 : Outport  Port=11
  Out12 : Outport  Port=12
  wires:
  B/1 -> " Comparator Phase B"/1(Ref signal)
  SPWM A/2(Out2) -> Out2/1
  SPWM A/3(Out3) -> Out3/1
  SPWM A/1(Out1) -> Out1/1
  SPWM A/4(Out4) -> Out4/1
  C/1 -> Comparator Phase C/1(Ref Signal)
  Comparator Phase C/1(Out1) -> SPWM C/1(In1), Scope3/1
  SPWM C/3(Out3) -> Out11/1
  SPWM C/2(Out2) -> Out10/1
  SPWM C/4(Out4) -> Out12/1
  SPWM C/1(Out1) -> Out9/1
  SPWM B/2(Out2) -> Out6/1, Scope4/2
  SPWM B/3(Out3) -> Out7/1, Scope4/3
  SPWM B/4(Out4) -> Out8/1, Scope4/4
  SPWM B/1(Out1) -> Out5/1, Scope4/1
  " Comparator Phase B"/1(Out1) -> Scope2/1, SPWM B/1(In1)
  A/1 -> Comparator Phase A/1("Ref Signal ")
  Comparator Phase A/1(Out1) -> SPWM A/1(Switching signal), Scope1/1

== system transfer_function_calculation/Generator/Generator /Inverse Clarke Transformation ==
  ab : Inport
  Demux : Demux  Outputs=2
  Gain1 : Gain  Gain=1/2
  Gain2 : Gain  Gain=sqrt(3)
  Gain4 : Gain  Gain=1/2
  Mux : Mux  Inputs=3
  Sum : Sum  Inputs=|-+
  Sum1 : Sum  Inputs=|--
  abc : Outport
  wires:
  Mux/1 -> abc/1
  ab/1 -> Demux/1
  Sum1/1 -> Gain1/1
  Sum/1 -> Gain4/1
  Gain2/1 -> Sum1/2, Sum/2
  Demux/1 -> Sum1/1, Sum/1, Mux/1
  Demux/2 -> Gain2/1
  Gain4/1 -> Mux/2
  Gain1/1 -> Mux/3

== system transfer_function_calculation/Generator/Generator /Inverse Park Transformation ==
  dq : Inport
  angle : Inport  Port=2
  Demux : Demux  Outputs=2
  Mux : Mux  Inputs=2
  Product{,1..3} (4 alike) : Product  RndMeth=Zero
  Sum : Sum  Inputs=|+-
  Sum1 : Sum  Inputs=|++
  cosine : Trigonometry  Operator=cos
  sine : Trigonometry
  ab : Outport
  wires:
  Sum1/1 -> Mux/2
  Sum/1 -> Mux/1
  Product2/1 -> Sum/2
  Product1/1 -> Sum/1
  Product3/1 -> Sum1/2
  Product/1 -> Sum1/1
  cosine/1 -> Product3/2, Product1/2
  sine/1 -> Product2/2, Product/2
  Demux/2 -> Product3/1, Product2/1
  Demux/1 -> Product1/1, Product/1
  Mux/1 -> ab/1
  dq/1 -> Demux/1
  angle/1 -> cosine/1, sine/1

== system transfer_function_calculation/Generator/Generator /PMS-model ==
  w : Inport
  Vd : Inport  Port=2
  Vq : Inport  Port=3
  1/Ld : Gain  Gain=1/Ld
  1/Lq : Gain  Gain=1/Lq
  3/2 p : Gain  Gain=3/2*p
  "Flux " : Gain  Gain=Flux
  Flux 1 : Gain  Gain=Flux
  Integrator : Integrator
  Integrator1 : Integrator
  Ld : Gain  Gain=Ld
  Ld-Lq : Gain  Gain=Ld-Lq
  Lq : Gain  Gain=Lq
  Mux : Mux  Inputs=2
  Product : Product
  Product1 : Product
  Product2 : Product
  R : Gain  Gain=Rs
  R1 : Gain  Gain=Rs
  Sum : Sum  Inputs=|+-+
  Sum1 : Sum  Inputs=|---+
  Sum3 : Sum  Inputs=|++
  Torque : Outport
  I_dq : Outport  Port=2
  wires:
  R/1 -> Sum/2
  Product1/1 -> Sum1/1
  w/1 -> "Flux "/1, Product1/1, Product/1
  Vd/1 -> Sum/3
  3/2 p/1 -> Torque/1
  Mux/1 -> I_dq/1
  Product/1 -> Sum/1
  Sum3/1 -> 3/2 p/1
  R1/1 -> Sum1/2
  Sum/1 -> 1/Ld/1
  1/Ld/1 -> Integrator/1
  Integrator/1 -> Product2/1, R/1, Ld/1, Mux/1
  Sum1/1 -> 1/Lq/1
  1/Lq/1 -> Integrator1/1
  Integrator1/1 -> Product2/2, Flux 1/1, R1/1, Lq/1, Mux/2
  Ld/1 -> Product1/2
  Lq/1 -> Product/2
  Vq/1 -> Sum1/4
  "Flux "/1 -> Sum1/3
  Flux 1/1 -> Sum3/1
  Ld-Lq/1 -> Sum3/2
  Product2/1 -> Ld-Lq/1

== system transfer_function_calculation/Generator/Generator /Parktransformation ==
  v_abc : Inport
  theta : Inport  Port=2
  Scope1 : Scope
  Scope2 : Scope
  Scope3 : Scope
  Three-phase current : Subsystem
  abc to alpha-beta : Subsystem
  alpha-beta to dq : Subsystem
  f : Constant  Value=50
  f1 : Constant  Value=20
  v_dq : Outport
  wires:
  abc to alpha-beta/1("alpha-beta ") -> Scope1/1, alpha-beta to dq/2("alpha-beta ")
  alpha-beta to dq/1(Out1) -> v_dq/1, Scope2/1
  f1/1 -> Three-phase current/2(In2)
  v_abc/1 -> Scope3/1, abc to alpha-beta/1(abc)
  theta/1 -> alpha-beta to dq/1(theta)
